simulink model "DCMotorFault_sim"  (R2019a)
settings: Solver=VariableStepAuto  StartTime=0.0  StopTime=simEnd  FixedStep=T  MaxStep=T  RelTol=1e-3
values from neighbouring files (symbols this model uses):
  Bm = 3e-3    (= 0.003)    [getMotorValues.m]
  Jm = 2.36e-2    (= 0.0236)    [getMotorValues.m]
  Kt = AddVariation(Kt,0.1)    [getMotorValues.m]
  La = AddVariation(La,0.05)    [getMotorValues.m]
  Ra = AddVariation(Ra,0.075)    [getMotorValues.m]
  T = 0.001    [DCMotorFault.m]    (also in GenerateMotorFault.m; GenerateMotorValues.m; SetupMotor.m)
  tBm = faultTime    [getFaultParam.m]
  tI = faultTime    [getFaultParam.m]
  tU = faultTime    [getFaultParam.m]
  tUt = faultTime    [getFaultParam.m]
  tW = faultTime    [getFaultParam.m]
settings Model: Creator=alexc  LastModifiedBy=alexc

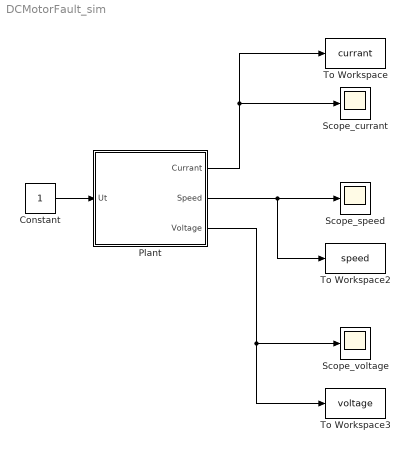
== system DCMotorFault_sim ==
  Constant : Constant
  Plant : Subsystem
  Scope_currant : Scope
  Scope_speed : Scope
  Scope_voltage : Scope
  To Workspace : ToWorkspace  VariableName=currant  SaveFormat=Timeseries  SampleTime=T
  To Workspace2 : ToWorkspace  VariableName=speed  SaveFormat=Timeseries  SampleTime=T
  To Workspace3 : ToWorkspace  VariableName=voltage  SaveFormat=Timeseries  SampleTime=T
  wires:
  Plant/2(Speed) -> To Workspace2/1, Scope_speed/1
  Plant/1(Currant) -> To Workspace/1, Scope_currant/1
  Plant/3(Voltage) -> Scope_voltage/1, To Workspace3/1
  Constant/1 -> Plant/1(Ut)

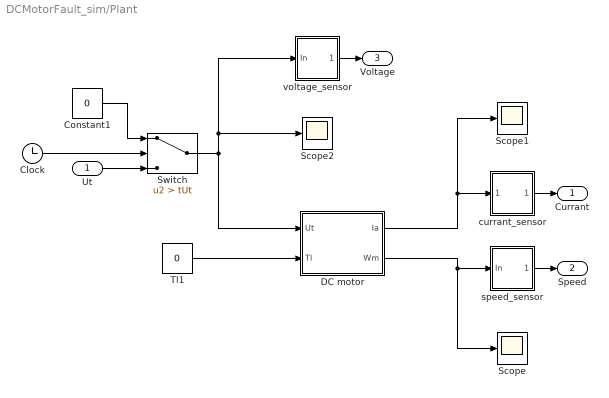
== system DCMotorFault_sim/Plant ==
  Ut : Inport
  Clock : Clock
  Constant1 : Constant  Value=0
  DC motor : Subsystem
  Scope : Scope
  Scope1 : Scope
  Scope2 : Scope
  Switch : Switch  Criteria=u2 > Threshold  Threshold=tUt
  Tl1 : Constant  Value=0
  currant_sensor : Subsystem
  speed_sensor : Subsystem
  voltage_sensor : Subsystem
  Currant : Outport
  Speed : Outport  Port=2
  Voltage : Outport  Port=3
  wires:
  Tl1/1 -> DC motor/2(Tl)
  speed_sensor/1(value) -> Speed/1
  DC motor/2(Wm) -> Scope/1, speed_sensor/1(In)
  currant_sensor/1(value) -> Currant/1
  DC motor/1(Ia) -> currant_sensor/1(In1), Scope1/1
  Switch/1 -> DC motor/1(Ut), Scope2/1, voltage_sensor/1(In)
  Clock/1 -> Switch/2
  Constant1/1 -> Switch/1
  Ut/1 -> Switch/3
  voltage_sensor/1(value) -> Voltage/1

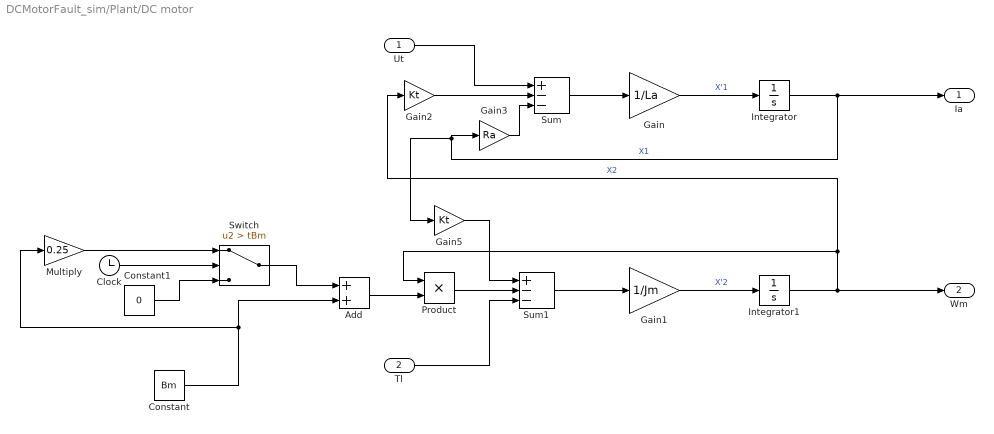
== system DCMotorFault_sim/Plant/DC motor ==
  Ut : Inport
  Tl : Inport  Port=2
  Add : Sum
  Clock : Clock
  Constant : Constant  Value=Bm
  Constant1 : Constant  Value=0
  Gain : Gain  Gain=1/La
  Gain1 : Gain  Gain=1/Jm
  Gain2 : Gain  Gain=Kt
  Gain3 : Gain  Gain=Ra
  Gain5 : Gain  Gain=Kt
  Integrator : Integrator
  Integrator1 : Integrator
  Multiply : Gain  Gain=0.25
  Product : Product
  Sum : Sum  Inputs=+--
  Sum1 : Sum  Inputs=+--
  Switch : Switch  Criteria=u2 > Threshold  Threshold=tBm
  Ia : Outport
  Wm : Outport  Port=2
  wires:
  Gain/1 -> Integrator/1  "X'1"
  Sum/1 -> Gain/1
  Integrator/1 -> Gain5/1, Gain3/1, Ia/1  "X1"
  Integrator1/1 -> Product/1, Gain2/1, Wm/1  "X2"
  Sum1/1 -> Gain1/1
  Gain1/1 -> Integrator1/1  "X'2"
  Ut/1 -> Sum/1
  Gain2/1 -> Sum/2
  Gain3/1 -> Sum/3
  Tl/1 -> Sum1/3
  Product/1 -> Sum1/2
  Gain5/1 -> Sum1/1
  Constant/1 -> Multiply/1, Add/2
  Clock/1 -> Switch/2
  Switch/1 -> Add/1
  Add/1 -> Product/2
  Constant1/1 -> Switch/3
  Multiply/1 -> Switch/1

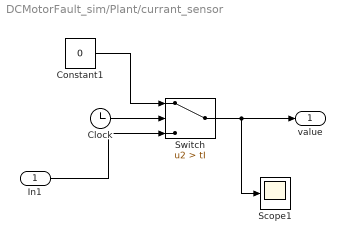
== system DCMotorFault_sim/Plant/currant_sensor ==
  In1 : Inport
  Clock : Clock
  Constant1 : Constant  Value=0
  Scope1 : Scope
  Switch : Switch  Criteria=u2 > Threshold  Threshold=tI
  value : Outport
  wires:
  Clock/1 -> Switch/2
  Constant1/1 -> Switch/1
  Switch/1 -> Scope1/1, value/1
  In1/1 -> Switch/3

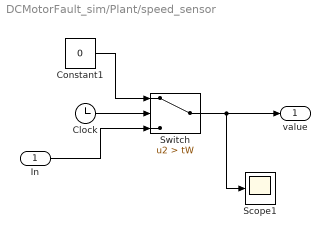
== system DCMotorFault_sim/Plant/speed_sensor ==
  In : Inport
  Clock : Clock
  Constant1 : Constant  Value=0
  Scope1 : Scope
  Switch : Switch  Criteria=u2 > Threshold  Threshold=tW
  value : Outport
  wires:
  Clock/1 -> Switch/2
  Constant1/1 -> Switch/1
  Switch/1 -> Scope1/1, value/1
  In/1 -> Switch/3

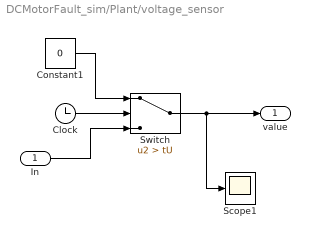
== system DCMotorFault_sim/Plant/voltage_sensor ==
  In : Inport
  Clock : Clock
  Constant1 : Constant  Value=0
  Scope1 : Scope
  Switch : Switch  Criteria=u2 > Threshold  Threshold=tU
  value : Outport
  wires:
  Clock/1 -> Switch/2
  Constant1/1 -> Switch/1
  Switch/1 -> Scope1/1, value/1
  In/1 -> Switch/3
